simulink model "ODE"  (R2016a)
settings: Solver=ode1  StartTime=0.0  StopTime=10.0  FixedStep=0.01  RelTol=1e-3
settings Model: Creator=chris.barlow  LastModifiedBy=chris.barlow

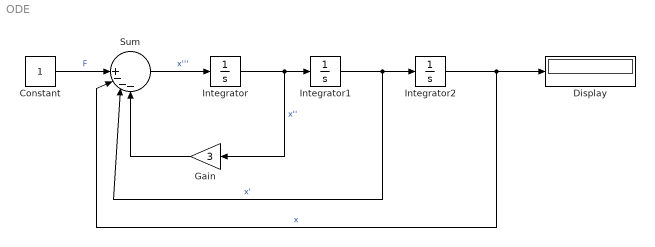
== system ODE ==
  Constant : Constant
  Display : Display
  Gain : Gain  Gain=3
  Integrator : Integrator  InitialCondition=3
  Integrator1 : Integrator  InitialCondition=2
  Integrator2 : Integrator  InitialCondition=1
  Sum : Sum  Inputs=|||+---
  wires:
  Sum/1 -> Integrator/1  "x'''"
  Integrator/1 -> Gain/1, Integrator1/1  "x''"
  Integrator1/1 -> Integrator2/1, Sum/3  "x'"
  Integrator2/1 -> Display/1, Sum/2  "x"
  Constant/1 -> Sum/1  "F"
  Gain/1 -> Sum/4
